simulink subsystem "suspensionOneDOF"  (R2023a)
settings: Solver=VariableStepAuto  StartTime=0.0  StopTime=10.0  RelTol=1e-3
model mask{obj=obj}
  mask prompts: obj "Part Object:"
settings Model: Creator=grouleau  LastModifiedBy=grouleau

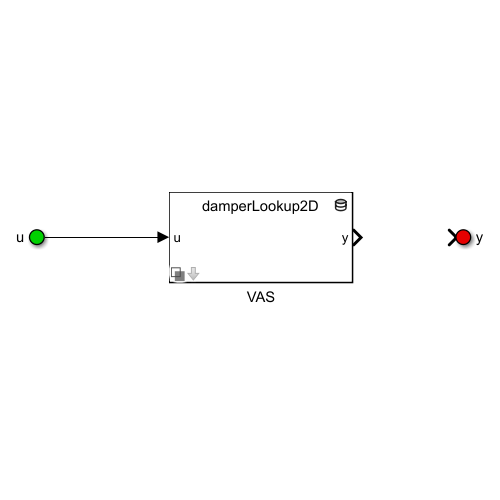
[thumbnail: Simulink's stored preview of the top-level diagram]
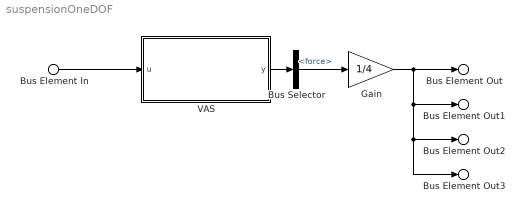
== system suspensionOneDOF ==
  Bus Element In : Inport  PortName=u  Element=FrontRight
  Bus Selector : BusSelector  OutputSignals=force
  Gain : Gain  Gain=1/4
  VAS : Subsystem  Variant=on  VariantChoicesSpecifier=obj.getVariantChoices()  VariantControlMode=label  LabelModeActiveChoice=suspension  mask{obj=obj.Suspension}
      mask prompts: obj "Part Object"
  Bus Element Out : Outport  PortName=y  Element=Forces.FrontRight
  Bus Element Out1 : Outport  PortName=y  Element=Forces.FrontLeft
  Bus Element Out2 : Outport  PortName=y  Element=Forces.RearRight
  Bus Element Out3 : Outport  PortName=y  Element=Forces.RearLeft
  wires:
  Bus Element In/1 -> VAS/1(u)
  VAS/1(y) -> Bus Selector/1
  Gain/1 -> Bus Element Out/1, Bus Element Out1/1, Bus Element Out3/1, Bus Element Out2/1
  Bus Selector/1 -> Gain/1  "<force>"

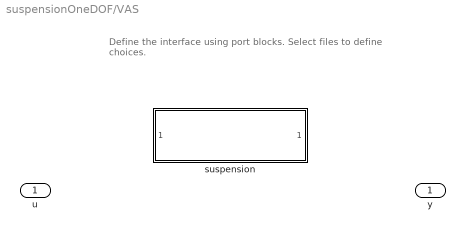
== system suspensionOneDOF/VAS ==
  note: Define the interface using port blocks.
      | Select files to define choices.
  u : Inport
  suspension : Subsystem  VariantControl=suspension  ReferencedSubsystem=suspension  obj=obj
  y : Outport
